simulink model "power_10MW5_diode"  (R2023b)
settings: Solver=FixedStepDiscrete  StartTime=0.0  StopTime=2.6  RelTol=1e-3
InitFcn:
  | power_sysinit
StopFcn:
  | ans = [pl_T1(end),max(tem_T1),pl_T2(end),max(tem_T2),pl_D1(end),max(tem_D1),...
  |     pl_D2(end),max(tem_D2),pl_D5(end),max(tem_D5),i_45(end),i_15(end),pl_D7(end),max(tem_D7)]
values from neighbouring files (symbols this model uses):
  C_absorption = 34e-6    (= 3.4e-05)    [power_sysinit.m]
  f = 40    [power_sysinit.m]
  f_switch = 900    [power_sysinit.m]
  IN = 0.3    [power_sysinit.m]
  L_absorption = 4e-6    (= 4e-06)    [power_sysinit.m]
  m = 1/75*f    (= 0.533333333333)    [power_sysinit.m]
  PM = 0    [power_sysinit.m]
  R_absorption = 0.45    [power_sysinit.m]
  TC = 1/f_switch    (= 0.00111111111111)    [power_sysinit.m]
  temp_init = 40    [power_sysinit.m]
  Ts1 = 1e-6    (= 1e-06)    [power_sysinit.m]
  Ts2 = 500E-6    (= 0.0005)    [power_sysinit.m]
  Udc = 2500    [power_sysinit.m]
undefined symbols (not defined in the file or in its folder): DIODE_204520, DIODE_344520, DIODE_364520, DIODE_364521, DIODE_D1031SH, DIODE_D1331SH, IGCT_364520_36, IGCT_364521_36, IGCT_654522_6, magnitude, Rth_h, Rth_h_tau
libraries: spsMeanLib x138, simulink x32, spsSeriesRLCBranchLib x30, spsRMSLib x24, spsCurrentMeasurementLib x21, dspstat3 x13, spsDiodeLib x12, spsVoltageMeasurementLib x12, spsOnDelayLib x6, powerlib_extras x5, spsDCVoltageSourceLib x4, spsIGBTDiodeLib x4
(part 5 of 6)

== system power_10MW5_diode/JUNCTION LOSS and TEMP/DIODE/36L4521_D/36l4521_MAIN/Subsystem34 ==
  In1 : Inport
  In2 : Inport  Port=2
  In3 : Inport  Port=3
  Abs1 : Abs  SaturateOnIntegerOverflow=off
  Add : Sum
  Constant1 : Constant  Value=0
  Constant2 : Constant  Value=0
  Gain2 : Gain  Gain=Udc/DIODE_364521.Vdc
  Gain3 : Gain  Gain=1/Ts2
  Gain4 : Gain
  Gain8 : Gain  Gain=DIODE_364521.Err/DIODE_364521.IFQ
  Logical Operator1 : Logic  Operator=NOT  AllPortsSameDT=off  OutDataTypeStr=boolean
  Logical Operator11 : Logic  Operator=OR  AllPortsSameDT=off  OutDataTypeStr=boolean
  Logical Operator2 : Logic  Operator=NOT  AllPortsSameDT=off  OutDataTypeStr=boolean
  Logical Operator3 : Logic  AllPortsSameDT=off  OutDataTypeStr=boolean
  Logical Operator4 : Logic  AllPortsSameDT=off  OutDataTypeStr=boolean
  Logical Operator5 : Logic  Operator=NOT  AllPortsSameDT=off  OutDataTypeStr=boolean
  Logical Operator6 : Logic  AllPortsSameDT=off  OutDataTypeStr=boolean
  Pulse Generator : DiscretePulseGenerator  PulseType=Time based  Period=Ts2  PulseWidth=5
  Saturation : Saturate  UpperLimit=5500  LowerLimit=0
  Saturation1 : Saturate  UpperLimit=100  LowerLimit=0
  Scope1 : Scope  NumInputPorts=3
  Scope7 : Scope  NumInputPorts=2
  Switch2 : Switch  Criteria=u2 > Threshold  SaturateOnIntegerOverflow=off  InputSameDT=off
  Switch3 : Switch  Criteria=u2 > Threshold  SaturateOnIntegerOverflow=off  InputSameDT=off
  Switch4 : Switch  Criteria=u2 > Threshold  SaturateOnIntegerOverflow=off  InputSameDT=off
  Unit Delay{,1..4} (5 alike) : UnitDelay  SampleTime=1e-6  HasFrameUpgradeWarning=on
  Out1 : Outport  VectorParamsAs1DForOutWhenUnconnected=off
  wires:
  Abs1/1 -> Add/1
  Switch2/1 -> Gain2/1
  Gain2/1 -> Abs1/1, Scope1/1
  In2/1 -> Logical Operator3/1, Unit Delay/1
  Logical Operator2/1 -> Logical Operator3/2
  Constant2/1 -> Switch2/3
  Switch3/1 -> Add/2
  Constant1/1 -> Switch3/1
  Pulse Generator/1 -> Unit Delay3/1, Logical Operator4/1
  Switch4/1 -> Scope7/2, Gain3/1, Unit Delay2/1
  Unit Delay2/1 -> Switch4/3
  Unit Delay3/1 -> Logical Operator5/1
  Logical Operator5/1 -> Logical Operator4/2
  Logical Operator4/1 -> Switch4/2, Switch3/2, Scope1/3
  Unit Delay1/1 -> Scope7/1, Switch4/1, Switch3/3
  Gain3/1 -> Out1/1
  In1/1 -> Gain4/1
  Add/1 -> Scope1/2, Unit Delay1/1
  Unit Delay/1 -> Logical Operator2/1
  Gain4/1 -> Saturation/1
  Saturation1/1 -> Switch2/1
  In3/1 -> Unit Delay4/1, Logical Operator6/1
  Unit Delay4/1 -> Logical Operator1/1
  Logical Operator6/1 -> Logical Operator11/2
  Logical Operator1/1 -> Logical Operator6/2
  Logical Operator11/1 -> Switch2/2
  Logical Operator3/1 -> Logical Operator11/1
  Saturation/1 -> Gain8/1
  Gain8/1 -> Saturation1/1

== system power_10MW5_diode/JUNCTION LOSS and TEMP/DIODE/36L4521_D/36l4521_MAIN/Subsystem4 ==
  note: 接触热阻：散热器到壳
      | 需考虑单面散热还是双面
      | 时间常数估计的？
  note: 器件手册热阻：壳到结
  note: 散热器热阻：水到壳
  In1 : Inport
  In2 : Inport  Port=2
  Add3 : Sum
  Add4 : Sum  Inputs=5
  Add5 : Sum  Inputs=+++
  Constant : Constant  Value=temp_init
  Discrete Filter1 : DiscreteFilter  Numerator=[Ts2/DIODE_364521.Rth_jc1_dou_tau]  Denominator=[1 (Ts2/DIODE_364521.Rth_jc1_dou_tau)-1]  SampleTime=Ts2
  Discrete Filter2 : DiscreteFilter  Numerator=[Ts2/DIODE_364521.Rth_jc2_dou_tau]  Denominator=[1 (Ts2/DIODE_364521.Rth_jc2_dou_tau)-1]  SampleTime=Ts2
  Discrete Filter3 : DiscreteFilter  Numerator=[Ts2/DIODE_364521.Rth_jc3_dou_tau]  Denominator=[1 (Ts2/DIODE_364521.Rth_jc3_dou_tau)-1]  SampleTime=Ts2
  Discrete Filter4 : DiscreteFilter  Numerator=[Ts2/DIODE_364521.Rth_jc4_dou_tau]  Denominator=[1 (Ts2/DIODE_364521.Rth_jc4_dou_tau)-1]  SampleTime=Ts2
  Discrete Filter5 : DiscreteFilter  Numerator=[Ts2/DIODE_364521.Rth_ch_dou_tau]  Denominator=[1 (Ts2/DIODE_364521.Rth_ch_dou_tau)-1]  SampleTime=Ts2
  Discrete Filter9 : DiscreteFilter  Numerator=[Ts2/Rth_h_tau]  Denominator=[1 (Ts2/Rth_h_tau)-1]  SampleTime=Ts2
  Gain1 : Gain  Gain=DIODE_364521.Rth_jc1_dou
  Gain2 : Gain  Gain=DIODE_364521.Rth_jc2_dou
  Gain3 : Gain  Gain=DIODE_364521.Rth_jc3_dou
  Gain4 : Gain  Gain=DIODE_364521.Rth_jc4_dou
  Gain5 : Gain  Gain=DIODE_364521.Rth_ch_dou
  Gain9 : Gain  Gain=Rth_h
  Out1 : Outport  VectorParamsAs1DForOutWhenUnconnected=off
  wires:
  Discrete Filter9/1 -> Add5/1
  Gain9/1 -> Discrete Filter9/1
  Add3/1 -> Gain2/1, Gain1/1, Gain9/1, Gain4/1, Gain5/1, Gain3/1
  Discrete Filter3/1 -> Add4/4
  Gain3/1 -> Discrete Filter3/1
  Discrete Filter5/1 -> Add4/1
  Gain5/1 -> Discrete Filter5/1
  Discrete Filter1/1 -> Add4/2
  Add5/1 -> Out1/1
  Gain1/1 -> Discrete Filter1/1
  Constant/1 -> Add5/3
  In2/1 -> Add3/2
  Add4/1 -> Add5/2
  Discrete Filter2/1 -> Add4/3
  Gain2/1 -> Discrete Filter2/1
  In1/1 -> Add3/1
  Gain4/1 -> Discrete Filter4/1
  Discrete Filter4/1 -> Add4/5

== system power_10MW5_diode/JUNCTION LOSS and TEMP/DIODE/36L4521_D/36l4521_MAIN/Subsystem5 ==
  In1 : Inport
  Gain44 : Gain  Gain=DIODE_364521.rF
  Gain45 : Gain  Gain=DIODE_364521.VF0
  Math Function9 : Math  Operator=magnitude^2  SignedPower=on
  Mean79 : spsMeanLib/Mean  Freq=2000  Vinit=0  Ts=Ts1
  RMS9 : spsRMSLib/RMS  TrueRMS=on  Freq=2000  RMSInit=0  Ts=Ts1
  Out1 : Outport
  Out2 : Outport  Port=2
  wires:
  Gain45/1 -> Out2/1
  In1/1 -> RMS9/1, Mean79/1
  Math Function9/1 -> Gain44/1
  Mean79/1 -> Gain45/1
  Gain44/1 -> Out1/1
  RMS9/1 -> Math Function9/1

== system power_10MW5_diode/JUNCTION LOSS and TEMP/DIODE/36L4521_D/36l4521_MAIN/Subsystem53 ==
  note: 散热器热阻：水到壳
  note: 器件手册热阻：壳到结
  note: 接触热阻：散热器到壳
      | 需考虑单面散热还是双面
      | 时间常数估计的？
  In1 : Inport
  In2 : Inport  Port=2
  Add3 : Sum
  Add4 : Sum  Inputs=5
  Add5 : Sum  Inputs=+++
  Constant : Constant  Value=temp_init
  Discrete Filter1 : DiscreteFilter  Numerator=[Ts2/DIODE_364521.Rth_jc1_dou_tau]  Denominator=[1 (Ts2/DIODE_364521.Rth_jc1_dou_tau)-1]  SampleTime=Ts2
  Discrete Filter2 : DiscreteFilter  Numerator=[Ts2/DIODE_364521.Rth_jc2_dou_tau]  Denominator=[1 (Ts2/DIODE_364521.Rth_jc2_dou_tau)-1]  SampleTime=Ts2
  Discrete Filter3 : DiscreteFilter  Numerator=[Ts2/DIODE_364521.Rth_jc3_dou_tau]  Denominator=[1 (Ts2/DIODE_364521.Rth_jc3_dou_tau)-1]  SampleTime=Ts2
  Discrete Filter4 : DiscreteFilter  Numerator=[Ts2/DIODE_364521.Rth_jc4_dou_tau]  Denominator=[1 (Ts2/DIODE_364521.Rth_jc4_dou_tau)-1]  SampleTime=Ts2
  Discrete Filter5 : DiscreteFilter  Numerator=[Ts2/DIODE_364521.Rth_ch_dou_tau]  Denominator=[1 (Ts2/DIODE_364521.Rth_ch_dou_tau)-1]  SampleTime=Ts2
  Discrete Filter9 : DiscreteFilter  Numerator=[Ts2/Rth_h_tau]  Denominator=[1 (Ts2/Rth_h_tau)-1]  SampleTime=Ts2
  Gain1 : Gain  Gain=DIODE_364521.Rth_jc1_dou
  Gain2 : Gain  Gain=DIODE_364521.Rth_jc2_dou
  Gain3 : Gain  Gain=DIODE_364521.Rth_jc3_dou
  Gain4 : Gain  Gain=DIODE_364521.Rth_jc4_dou
  Gain5 : Gain  Gain=DIODE_364521.Rth_ch_dou
  Gain9 : Gain  Gain=Rth_h
  Out1 : Outport  VectorParamsAs1DForOutWhenUnconnected=off
  wires:
  Discrete Filter4/1 -> Add4/5
  Gain4/1 -> Discrete Filter4/1
  In1/1 -> Add3/1
  Gain2/1 -> Discrete Filter2/1
  Discrete Filter2/1 -> Add4/3
  Add4/1 -> Add5/2
  In2/1 -> Add3/2
  Constant/1 -> Add5/3
  Gain1/1 -> Discrete Filter1/1
  Add5/1 -> Out1/1
  Discrete Filter1/1 -> Add4/2
  Gain5/1 -> Discrete Filter5/1
  Discrete Filter5/1 -> Add4/1
  Gain3/1 -> Discrete Filter3/1
  Discrete Filter3/1 -> Add4/4
  Add3/1 -> Gain3/1, Gain5/1, Gain4/1, Gain9/1, Gain1/1, Gain2/1
  Gain9/1 -> Discrete Filter9/1
  Discrete Filter9/1 -> Add5/1

== system power_10MW5_diode/JUNCTION LOSS and TEMP/DIODE/36L4521_D/36l4521_MAIN/Subsystem6 ==
  note: 用于判断D1关断时刻，电流为负时，T3开通就意味着D1关断
  In1 : Inport
  In2 : Inport  Port=2
  Abs1 : Abs  SaturateOnIntegerOverflow=off
  Add : Sum
  Constant1 : Constant  Value=0
  Constant2 : Constant  Value=0
  Gain1 : Gain  Gain=Udc/DIODE_364521.Vdc
  Gain2 : Gain  Gain=DIODE_364521.Err/DIODE_364521.IFQ
  Gain3 : Gain  Gain=1/Ts2
  Gain4 : Gain
  Logical Operator2 : Logic  Operator=NOT  AllPortsSameDT=off  OutDataTypeStr=boolean
  Logical Operator3 : Logic  AllPortsSameDT=off  OutDataTypeStr=boolean
  Logical Operator4 : Logic  AllPortsSameDT=off  OutDataTypeStr=boolean
  Logical Operator5 : Logic  Operator=NOT  AllPortsSameDT=off  OutDataTypeStr=boolean
  Pulse Generator : DiscretePulseGenerator  PulseType=Time based  Period=Ts2  PulseWidth=5
  Saturation : Saturate  UpperLimit=5500  LowerLimit=0
  Saturation1 : Saturate  UpperLimit=100  LowerLimit=0
  Switch2 : Switch  Criteria=u2 > Threshold  SaturateOnIntegerOverflow=off  InputSameDT=off
  Switch3 : Switch  Criteria=u2 > Threshold  SaturateOnIntegerOverflow=off  InputSameDT=off
  Switch4 : Switch  Criteria=u2 > Threshold  SaturateOnIntegerOverflow=off  InputSameDT=off
  Unit Delay{,1..3} (4 alike) : UnitDelay  SampleTime=Ts1  HasFrameUpgradeWarning=on
  Out1 : Outport  VectorParamsAs1DForOutWhenUnconnected=off
  wires:
  Gain2/1 -> Saturation1/1
  Saturation/1 -> Gain2/1
  Saturation1/1 -> Switch2/1
  Gain4/1 -> Saturation/1
  Unit Delay/1 -> Logical Operator2/1
  Add/1 -> Unit Delay1/1
  In1/1 -> Gain4/1
  Gain3/1 -> Out1/1
  Unit Delay1/1 -> Switch4/1, Switch3/3
  Logical Operator4/1 -> Switch3/2, Switch4/2
  Logical Operator5/1 -> Logical Operator4/2
  Unit Delay3/1 -> Logical Operator5/1
  Unit Delay2/1 -> Switch4/3
  Switch4/1 -> Gain3/1, Unit Delay2/1
  Pulse Generator/1 -> Logical Operator4/1, Unit Delay3/1
  Constant1/1 -> Switch3/1
  Switch3/1 -> Add/2
  Constant2/1 -> Switch2/3
  Logical Operator3/1 -> Switch2/2
  Logical Operator2/1 -> Logical Operator3/2
  In2/1 -> Unit Delay/1, Logical Operator3/1
  Gain1/1 -> Abs1/1
  Switch2/1 -> Gain1/1
  Abs1/1 -> Add/1

== system power_10MW5_diode/JUNCTION LOSS and TEMP/DIODE/36L4521_D/36l4521_MAIN/Subsystem7 ==
  note: 散热器热阻：水到壳
  note: 器件手册热阻：壳到结
  note: 接触热阻：散热器到壳
      | 需考虑单面散热还是双面
      | 时间常数估计的？
  In1 : Inport
  In2 : Inport  Port=2
  Add3 : Sum
  Add4 : Sum  Inputs=5
  Add5 : Sum  Inputs=+++
  Constant : Constant  Value=temp_init
  Discrete Filter1 : DiscreteFilter  Numerator=[Ts2/DIODE_364521.Rth_jc1_dou_tau]  Denominator=[1 (Ts2/DIODE_364521.Rth_jc1_dou_tau)-1]  SampleTime=Ts2
  Discrete Filter2 : DiscreteFilter  Numerator=[Ts2/DIODE_364521.Rth_jc2_dou_tau]  Denominator=[1 (Ts2/DIODE_364521.Rth_jc2_dou_tau)-1]  SampleTime=Ts2
  Discrete Filter3 : DiscreteFilter  Numerator=[Ts2/DIODE_364521.Rth_jc3_dou_tau]  Denominator=[1 (Ts2/DIODE_364521.Rth_jc3_dou_tau)-1]  SampleTime=Ts2
  Discrete Filter4 : DiscreteFilter  Numerator=[Ts2/DIODE_364521.Rth_jc4_dou_tau]  Denominator=[1 (Ts2/DIODE_364521.Rth_jc4_dou_tau)-1]  SampleTime=Ts2
  Discrete Filter5 : DiscreteFilter  Numerator=[Ts2/DIODE_364521.Rth_ch_dou_tau]  Denominator=[1 (Ts2/DIODE_364521.Rth_ch_dou_tau)-1]  SampleTime=Ts2
  Discrete Filter9 : DiscreteFilter  Numerator=[Ts2/Rth_h_tau]  Denominator=[1 (Ts2/Rth_h_tau)-1]  SampleTime=Ts2
  Gain1 : Gain  Gain=DIODE_364521.Rth_jc1_dou
  Gain2 : Gain  Gain=DIODE_364521.Rth_jc2_dou
  Gain3 : Gain  Gain=DIODE_364521.Rth_jc3_dou
  Gain4 : Gain  Gain=DIODE_364521.Rth_jc4_dou
  Gain5 : Gain  Gain=DIODE_364521.Rth_ch_dou
  Gain9 : Gain  Gain=Rth_h
  Out1 : Outport  VectorParamsAs1DForOutWhenUnconnected=off
  wires:
  Discrete Filter4/1 -> Add4/5
  Gain4/1 -> Discrete Filter4/1
  In1/1 -> Add3/1
  Gain2/1 -> Discrete Filter2/1
  Discrete Filter2/1 -> Add4/3
  Add4/1 -> Add5/2
  In2/1 -> Add3/2
  Constant/1 -> Add5/3
  Gain1/1 -> Discrete Filter1/1
  Add5/1 -> Out1/1
  Discrete Filter1/1 -> Add4/2
  Gain5/1 -> Discrete Filter5/1
  Discrete Filter5/1 -> Add4/1
  Gain3/1 -> Discrete Filter3/1
  Discrete Filter3/1 -> Add4/4
  Add3/1 -> Gain3/1, Gain5/1, Gain4/1, Gain9/1, Gain1/1, Gain2/1
  Gain9/1 -> Discrete Filter9/1
  Discrete Filter9/1 -> Add5/1

== system power_10MW5_diode/JUNCTION LOSS and TEMP/DIODE/36L4521_D/36l4521_MAIN/Subsystem8 ==
  In1 : Inport
  Gain44 : Gain  Gain=DIODE_364521.rF
  Gain45 : Gain  Gain=DIODE_364521.VF0
  Math Function9 : Math  Operator=magnitude^2  SignedPower=on
  Mean79 : spsMeanLib/Mean  Freq=2000  Vinit=0  Ts=Ts1
  RMS9 : spsRMSLib/RMS  TrueRMS=on  Freq=2000  RMSInit=0  Ts=Ts1
  Out1 : Outport
  Out2 : Outport  Port=2
  wires:
  RMS9/1 -> Math Function9/1
  Gain44/1 -> Out1/1
  Mean79/1 -> Gain45/1
  Math Function9/1 -> Gain44/1
  In1/1 -> Mean79/1, RMS9/1
  Gain45/1 -> Out2/1

== system power_10MW5_diode/JUNCTION LOSS and TEMP/DIODE/D1031SH/D1031SH_MAIN/Subsystem ==
  In1 : Inport
  Gain44 : Gain  Gain=DIODE_D1031SH.rF
  Gain45 : Gain  Gain=DIODE_D1031SH.VF0
  Math Function9 : Math  Operator=magnitude^2  SignedPower=on
  Mean79 : spsMeanLib/Mean  Freq=2000  Vinit=0  Ts=Ts1
  RMS9 : spsRMSLib/RMS  TrueRMS=on  Freq=2000  RMSInit=0  Ts=Ts1
  Out1 : Outport
  Out2 : Outport  Port=2
  wires:
  RMS9/1 -> Math Function9/1
  Gain44/1 -> Out1/1
  Mean79/1 -> Gain45/1
  Math Function9/1 -> Gain44/1
  In1/1 -> Mean79/1, RMS9/1
  Gain45/1 -> Out2/1

== system power_10MW5_diode/JUNCTION LOSS and TEMP/DIODE/D1031SH/D1031SH_MAIN/Subsystem1 ==
  note: 接触热阻：散热器到壳
      | 需考虑单面散热还是双面
      | 时间常数估计的？
  note: 器件手册热阻：壳到结
  note: 散热器热阻：水到壳
  In1 : Inport
  In2 : Inport  Port=2
  Add3 : Sum
  Add4 : Sum  Inputs=6
  Add5 : Sum  Inputs=+++
  Constant : Constant  Value=temp_init
  Discrete Filter1 : DiscreteFilter  Numerator=[Ts2/DIODE_D1031SH.Rth_jc1_dou_tau]  Denominator=[1 (Ts2/DIODE_D1031SH.Rth_jc1_dou_tau)-1]  SampleTime=Ts2
  Discrete Filter2 : DiscreteFilter  Numerator=[Ts2/DIODE_D1031SH.Rth_jc2_dou_tau]  Denominator=[1 (Ts2/DIODE_D1031SH.Rth_jc2_dou_tau)-1]  SampleTime=Ts2
  Discrete Filter3 : DiscreteFilter  Numerator=[Ts2/DIODE_D1031SH.Rth_jc3_dou_tau]  Denominator=[1 (Ts2/DIODE_D1031SH.Rth_jc3_dou_tau)-1]  SampleTime=Ts2
  Discrete Filter4 : DiscreteFilter  Numerator=[Ts2/DIODE_D1031SH.Rth_jc4_dou_tau]  Denominator=[1 (Ts2/DIODE_D1031SH.Rth_jc4_dou_tau)-1]  SampleTime=Ts2
  Discrete Filter5 : DiscreteFilter  Numerator=[Ts2/DIODE_D1031SH.Rth_ch_dou_tau]  Denominator=[1 (Ts2/DIODE_D1031SH.Rth_ch_dou_tau)-1]  SampleTime=Ts2
  Discrete Filter6 : DiscreteFilter  Numerator=[Ts2/DIODE_D1031SH.Rth_jc5_dou_tau]  Denominator=[1 (Ts2/DIODE_D1031SH.Rth_jc5_dou_tau)-1]  SampleTime=Ts2
  Discrete Filter9 : DiscreteFilter  Numerator=[Ts2/Rth_h_tau]  Denominator=[1 (Ts2/Rth_h_tau)-1]  SampleTime=Ts2
  Gain1 : Gain  Gain=DIODE_D1031SH.Rth_jc1_dou
  Gain2 : Gain  Gain=DIODE_D1031SH.Rth_jc2_dou
  Gain3 : Gain  Gain=DIODE_D1031SH.Rth_jc3_dou
  Gain4 : Gain  Gain=DIODE_D1031SH.Rth_jc4_dou
  Gain5 : Gain  Gain=DIODE_D1031SH.Rth_ch_dou
  Gain6 : Gain  Gain=DIODE_D1031SH.Rth_jc5_dou
  Gain9 : Gain  Gain=Rth_h
  Out1 : Outport  VectorParamsAs1DForOutWhenUnconnected=off
  wires:
  Discrete Filter6/1 -> Add4/6
  Gain6/1 -> Discrete Filter6/1
  Discrete Filter9/1 -> Add5/1
  Gain9/1 -> Discrete Filter9/1
  Add3/1 -> Gain2/1, Gain1/1, Gain9/1, Gain4/1, Gain6/1, Gain5/1, Gain3/1
  Discrete Filter3/1 -> Add4/4
  Gain3/1 -> Discrete Filter3/1
  Discrete Filter5/1 -> Add4/1
  Gain5/1 -> Discrete Filter5/1
  Discrete Filter1/1 -> Add4/2
  Add5/1 -> Out1/1
  Gain1/1 -> Discrete Filter1/1
  Constant/1 -> Add5/3
  In2/1 -> Add3/2
  Add4/1 -> Add5/2
  Discrete Filter2/1 -> Add4/3
  Gain2/1 -> Discrete Filter2/1
  In1/1 -> Add3/1
  Gain4/1 -> Discrete Filter4/1
  Discrete Filter4/1 -> Add4/5

== system power_10MW5_diode/JUNCTION LOSS and TEMP/DIODE/D1031SH/D1031SH_MAIN/Subsystem2 ==
  In1 : Inport
  Gain44 : Gain  Gain=DIODE_D1031SH.rF
  Gain45 : Gain  Gain=DIODE_D1031SH.VF0
  Math Function9 : Math  Operator=magnitude^2  SignedPower=on
  Mean79 : spsMeanLib/Mean  Freq=2000  Vinit=0  Ts=Ts1
  RMS9 : spsRMSLib/RMS  TrueRMS=on  Freq=2000  RMSInit=0  Ts=Ts1
  Out1 : Outport
  Out2 : Outport  Port=2
  wires:
  Gain45/1 -> Out2/1
  In1/1 -> RMS9/1, Mean79/1
  Math Function9/1 -> Gain44/1
  Mean79/1 -> Gain45/1
  Gain44/1 -> Out1/1
  RMS9/1 -> Math Function9/1

== system power_10MW5_diode/JUNCTION LOSS and TEMP/DIODE/D1031SH/D1031SH_MAIN/Subsystem29 ==
  note: 用于判断D1关断时刻，电流为负时，T3开通就意味着D1关断
  In1 : Inport
  In2 : Inport  Port=2
  Abs1 : Abs  SaturateOnIntegerOverflow=off
  Add : Sum
  Constant1 : Constant  Value=0
  Constant2 : Constant  Value=0
  Gain1 : Gain  Gain=Udc/DIODE_D1031SH.Vdc
  Gain2 : Gain  Gain=DIODE_D1031SH.Err/DIODE_D1031SH.IFQ
  Gain3 : Gain  Gain=1/Ts2
  Gain4 : Gain
  Logical Operator2 : Logic  Operator=NOT  AllPortsSameDT=off  OutDataTypeStr=boolean
  Logical Operator3 : Logic  AllPortsSameDT=off  OutDataTypeStr=boolean
  Logical Operator4 : Logic  AllPortsSameDT=off  OutDataTypeStr=boolean
  Logical Operator5 : Logic  Operator=NOT  AllPortsSameDT=off  OutDataTypeStr=boolean
  Pulse Generator : DiscretePulseGenerator  PulseType=Time based  Period=Ts2  PulseWidth=5
  Saturation : Saturate  UpperLimit=5500  LowerLimit=0
  Saturation1 : Saturate  UpperLimit=100  LowerLimit=0
  Switch2 : Switch  Criteria=u2 > Threshold  SaturateOnIntegerOverflow=off  InputSameDT=off
  Switch3 : Switch  Criteria=u2 > Threshold  SaturateOnIntegerOverflow=off  InputSameDT=off
  Switch4 : Switch  Criteria=u2 > Threshold  SaturateOnIntegerOverflow=off  InputSameDT=off
  Unit Delay{,1..3} (4 alike) : UnitDelay  SampleTime=Ts1  HasFrameUpgradeWarning=on
  Out1 : Outport  VectorParamsAs1DForOutWhenUnconnected=off
  wires:
  Abs1/1 -> Add/1
  Switch2/1 -> Gain1/1
  Gain1/1 -> Abs1/1
  In2/1 -> Logical Operator3/1, Unit Delay/1
  Logical Operator2/1 -> Logical Operator3/2
  Logical Operator3/1 -> Switch2/2
  Constant2/1 -> Switch2/3
  Switch3/1 -> Add/2
  Constant1/1 -> Switch3/1
  Pulse Generator/1 -> Unit Delay3/1, Logical Operator4/1
  Switch4/1 -> Unit Delay2/1, Gain3/1
  Unit Delay2/1 -> Switch4/3
  Unit Delay3/1 -> Logical Operator5/1
  Logical Operator5/1 -> Logical Operator4/2
  Logical Operator4/1 -> Switch4/2, Switch3/2
  Unit Delay1/1 -> Switch3/3, Switch4/1
  Gain3/1 -> Out1/1
  In1/1 -> Gain4/1
  Add/1 -> Unit Delay1/1
  Unit Delay/1 -> Logical Operator2/1
  Gain4/1 -> Saturation/1
  Saturation1/1 -> Switch2/1
  Saturation/1 -> Gain2/1
  Gain2/1 -> Saturation1/1

== system power_10MW5_diode/JUNCTION LOSS and TEMP/DIODE/D1031SH/D1031SH_MAIN/Subsystem3 ==
  In1 : Inport
  Abs1 : Abs  SaturateOnIntegerOverflow=off
  Add : Sum
  Add1 : Sum
  Constant : Constant
  Constant1 : Constant  Value=0
  Constant2 : Constant  Value=0
  Data Type Conversion : DataTypeConversion  OutDataTypeStr=boolean  SaturateOnIntegerOverflow=off  RndMeth=Floor
  Data Type Conversion1 : DataTypeConversion  SaturateOnIntegerOverflow=off  RndMeth=Floor
  Gain : Gain  Gain=-1
  Gain2 : Gain  Gain=Udc/DIODE_D1031SH.Vdc
  Gain3 : Gain  Gain=1/Ts2
  Gain6 : Gain
  Gain8 : Gain  Gain=DIODE_D1031SH.Err/DIODE_D1031SH.IFQ
  Logical Operator2 : Logic  Operator=NOT  AllPortsSameDT=off  OutDataTypeStr=boolean
  Logical Operator4 : Logic  AllPortsSameDT=off  OutDataTypeStr=boolean
  Logical Operator5 : Logic  Operator=NOT  AllPortsSameDT=off  OutDataTypeStr=boolean
  Pulse Generator : DiscretePulseGenerator  PulseType=Time based  Period=Ts2  PulseWidth=5
  Saturation2 : Saturate  UpperLimit=5500  LowerLimit=0
  Saturation3 : Saturate  UpperLimit=100  LowerLimit=0
  Scope1 : Scope  NumInputPorts=3
  Scope7 : Scope  NumInputPorts=2
  Switch2 : Switch  Criteria=u2 > Threshold  Threshold=-1  SaturateOnIntegerOverflow=off  InputSameDT=off
  Switch3 : Switch  Criteria=u2 > Threshold  SaturateOnIntegerOverflow=off  InputSameDT=off
  Switch4 : Switch  Criteria=u2 > Threshold  SaturateOnIntegerOverflow=off  InputSameDT=off
  Terminator : Terminator
  Unit Delay{,1..3} (4 alike) : UnitDelay  SampleTime=1e-6  HasFrameUpgradeWarning=on
  Out1 : Outport  VectorParamsAs1DForOutWhenUnconnected=off
  wires:
  Add/1 -> Unit Delay1/1, Scope1/2
  Gain3/1 -> Out1/1
  Unit Delay1/1 -> Switch4/1, Switch3/3, Scope7/1
  Logical Operator4/1 -> Switch3/2, Switch4/2, Scope1/3
  Logical Operator5/1 -> Logical Operator4/2
  Unit Delay3/1 -> Logical Operator5/1
  Unit Delay2/1 -> Switch4/3
  Switch4/1 -> Gain3/1, Unit Delay2/1, Scope7/2
  Pulse Generator/1 -> Logical Operator4/1, Unit Delay3/1
  Constant1/1 -> Switch3/1
  Switch3/1 -> Add/2
  Constant2/1 -> Switch2/3
  In1/1 -> Data Type Conversion/1, Gain6/1
  Gain2/1 -> Scope1/1, Abs1/1
  Switch2/1 -> Gain2/1
  Abs1/1 -> Add/1
  Unit Delay/1 -> Logical Operator2/1
  Logical Operator2/1 -> Add1/2
  Data Type Conversion/1 -> Add1/1, Unit Delay/1
  Add1/1 -> Data Type Conversion1/1
  Gain/1 -> Switch2/2
  Data Type Conversion1/1 -> Gain/1
  Constant/1 -> Switch2/1
  Gain6/1 -> Saturation2/1
  Saturation2/1 -> Gain8/1
  Gain8/1 -> Saturation3/1
  Saturation3/1 -> Terminator/1

== system power_10MW5_diode/JUNCTION LOSS and TEMP/DIODE/D1031SH/D1031SH_MAIN/Subsystem34 ==
  In1 : Inport
  In2 : Inport  Port=2
  In3 : Inport  Port=3
  Abs1 : Abs  SaturateOnIntegerOverflow=off
  Add : Sum
  Constant1 : Constant  Value=0
  Constant2 : Constant  Value=0
  Gain2 : Gain  Gain=Udc/DIODE_204520.Vdc
  Gain3 : Gain  Gain=1/Ts2
  Gain4 : Gain
  Gain8 : Gain  Gain=DIODE_D1031SH.Err/DIODE_D1031SH.IFQ
  Logical Operator1 : Logic  Operator=NOT  AllPortsSameDT=off  OutDataTypeStr=boolean
  Logical Operator11 : Logic  Operator=OR  AllPortsSameDT=off  OutDataTypeStr=boolean
  Logical Operator2 : Logic  Operator=NOT  AllPortsSameDT=off  OutDataTypeStr=boolean
  Logical Operator3 : Logic  AllPortsSameDT=off  OutDataTypeStr=boolean
  Logical Operator4 : Logic  AllPortsSameDT=off  OutDataTypeStr=boolean
  Logical Operator5 : Logic  Operator=NOT  AllPortsSameDT=off  OutDataTypeStr=boolean
  Logical Operator6 : Logic  AllPortsSameDT=off  OutDataTypeStr=boolean
  Pulse Generator : DiscretePulseGenerator  PulseType=Time based  Period=Ts2  PulseWidth=5
  Saturation : Saturate  UpperLimit=5500  LowerLimit=0
  Saturation1 : Saturate  UpperLimit=100  LowerLimit=0
  Scope1 : Scope  NumInputPorts=3
  Scope7 : Scope  NumInputPorts=2
  Switch2 : Switch  Criteria=u2 > Threshold  SaturateOnIntegerOverflow=off  InputSameDT=off
  Switch3 : Switch  Criteria=u2 > Threshold  SaturateOnIntegerOverflow=off  InputSameDT=off
  Switch4 : Switch  Criteria=u2 > Threshold  SaturateOnIntegerOverflow=off  InputSameDT=off
  Unit Delay{,1..4} (5 alike) : UnitDelay  SampleTime=1e-6  HasFrameUpgradeWarning=on
  Out1 : Outport  VectorParamsAs1DForOutWhenUnconnected=off
  wires:
  Abs1/1 -> Add/1
  Switch2/1 -> Gain2/1
  Gain2/1 -> Abs1/1, Scope1/1
  In2/1 -> Logical Operator3/1, Unit Delay/1
  Logical Operator2/1 -> Logical Operator3/2
  Constant2/1 -> Switch2/3
  Switch3/1 -> Add/2
  Constant1/1 -> Switch3/1
  Pulse Generator/1 -> Unit Delay3/1, Logical Operator4/1
  Switch4/1 -> Scope7/2, Gain3/1, Unit Delay2/1
  Unit Delay2/1 -> Switch4/3
  Unit Delay3/1 -> Logical Operator5/1
  Logical Operator5/1 -> Logical Operator4/2
  Logical Operator4/1 -> Switch4/2, Switch3/2, Scope1/3
  Unit Delay1/1 -> Scope7/1, Switch4/1, Switch3/3
  Gain3/1 -> Out1/1
  In1/1 -> Gain4/1
  Add/1 -> Scope1/2, Unit Delay1/1
  Unit Delay/1 -> Logical Operator2/1
  Gain4/1 -> Saturation/1
  Saturation1/1 -> Switch2/1
  In3/1 -> Unit Delay4/1, Logical Operator6/1
  Unit Delay4/1 -> Logical Operator1/1
  Logical Operator6/1 -> Logical Operator11/2
  Logical Operator1/1 -> Logical Operator6/2
  Logical Operator11/1 -> Switch2/2
  Logical Operator3/1 -> Logical Operator11/1
  Saturation/1 -> Gain8/1
  Gain8/1 -> Saturation1/1

== system power_10MW5_diode/JUNCTION LOSS and TEMP/DIODE/D1031SH/D1031SH_MAIN/Subsystem4 ==
  note: 接触热阻：散热器到壳
      | 需考虑单面散热还是双面
      | 时间常数估计的？
  note: 器件手册热阻：壳到结
  note: 散热器热阻：水到壳
  In1 : Inport
  In2 : Inport  Port=2
  Add3 : Sum
  Add4 : Sum  Inputs=6
  Add5 : Sum  Inputs=+++
  Constant : Constant  Value=temp_init
  Discrete Filter1 : DiscreteFilter  Numerator=[Ts2/DIODE_D1031SH.Rth_jc1_dou_tau]  Denominator=[1 (Ts2/DIODE_D1031SH.Rth_jc1_dou_tau)-1]  SampleTime=Ts2
  Discrete Filter2 : DiscreteFilter  Numerator=[Ts2/DIODE_D1031SH.Rth_jc2_dou_tau]  Denominator=[1 (Ts2/DIODE_D1031SH.Rth_jc2_dou_tau)-1]  SampleTime=Ts2
  Discrete Filter3 : DiscreteFilter  Numerator=[Ts2/DIODE_D1031SH.Rth_jc3_dou_tau]  Denominator=[1 (Ts2/DIODE_D1031SH.Rth_jc3_dou_tau)-1]  SampleTime=Ts2
  Discrete Filter4 : DiscreteFilter  Numerator=[Ts2/DIODE_D1031SH.Rth_jc4_dou_tau]  Denominator=[1 (Ts2/DIODE_D1031SH.Rth_jc4_dou_tau)-1]  SampleTime=Ts2
  Discrete Filter5 : DiscreteFilter  Numerator=[Ts2/DIODE_D1031SH.Rth_ch_dou_tau]  Denominator=[1 (Ts2/DIODE_D1031SH.Rth_ch_dou_tau)-1]  SampleTime=Ts2
  Discrete Filter6 : DiscreteFilter  Numerator=[Ts2/DIODE_D1031SH.Rth_jc5_dou_tau]  Denominator=[1 (Ts2/DIODE_D1031SH.Rth_jc5_dou_tau)-1]  SampleTime=Ts2
  Discrete Filter9 : DiscreteFilter  Numerator=[Ts2/Rth_h_tau]  Denominator=[1 (Ts2/Rth_h_tau)-1]  SampleTime=Ts2
  Gain1 : Gain  Gain=DIODE_D1031SH.Rth_jc1_dou
  Gain2 : Gain  Gain=DIODE_D1031SH.Rth_jc2_dou
  Gain3 : Gain  Gain=DIODE_D1031SH.Rth_jc3_dou
  Gain4 : Gain  Gain=DIODE_D1031SH.Rth_jc4_dou
  Gain5 : Gain  Gain=DIODE_D1031SH.Rth_ch_dou
  Gain6 : Gain  Gain=DIODE_D1031SH.Rth_jc5_dou
  Gain9 : Gain  Gain=Rth_h
  Out1 : Outport  VectorParamsAs1DForOutWhenUnconnected=off
  wires:
  Discrete Filter6/1 -> Add4/6
  Gain6/1 -> Discrete Filter6/1
  Discrete Filter9/1 -> Add5/1
  Gain9/1 -> Discrete Filter9/1
  Add3/1 -> Gain2/1, Gain1/1, Gain9/1, Gain4/1, Gain6/1, Gain5/1, Gain3/1
  Discrete Filter3/1 -> Add4/4
  Gain3/1 -> Discrete Filter3/1
  Discrete Filter5/1 -> Add4/1
  Gain5/1 -> Discrete Filter5/1
  Discrete Filter1/1 -> Add4/2
  Add5/1 -> Out1/1
  Gain1/1 -> Discrete Filter1/1
  Constant/1 -> Add5/3
  In2/1 -> Add3/2
  Add4/1 -> Add5/2
  Discrete Filter2/1 -> Add4/3
  Gain2/1 -> Discrete Filter2/1
  In1/1 -> Add3/1
  Gain4/1 -> Discrete Filter4/1
  Discrete Filter4/1 -> Add4/5

== system power_10MW5_diode/JUNCTION LOSS and TEMP/DIODE/D1031SH/D1031SH_MAIN/Subsystem5 ==
  In1 : Inport
  Gain44 : Gain  Gain=DIODE_D1031SH.rF
  Gain45 : Gain  Gain=DIODE_D1031SH.VF0
  Math Function9 : Math  Operator=magnitude^2  SignedPower=on
  Mean79 : spsMeanLib/Mean  Freq=2000  Vinit=0  Ts=Ts1
  RMS9 : spsRMSLib/RMS  TrueRMS=on  Freq=2000  RMSInit=0  Ts=Ts1
  Out1 : Outport
  Out2 : Outport  Port=2
  wires:
  RMS9/1 -> Math Function9/1
  Gain44/1 -> Out1/1
  Mean79/1 -> Gain45/1
  Math Function9/1 -> Gain44/1
  In1/1 -> Mean79/1, RMS9/1
  Gain45/1 -> Out2/1

== system power_10MW5_diode/JUNCTION LOSS and TEMP/DIODE/D1031SH/D1031SH_MAIN/Subsystem53 ==
  note: 散热器热阻：水到壳
  note: 器件手册热阻：壳到结
  note: 接触热阻：散热器到壳
      | 需考虑单面散热还是双面
      | 时间常数估计的？
  In1 : Inport
  In2 : Inport  Port=2
  Add3 : Sum
  Add4 : Sum  Inputs=6
  Add5 : Sum  Inputs=+++
  Constant : Constant  Value=temp_init
  Discrete Filter1 : DiscreteFilter  Numerator=[Ts2/DIODE_D1031SH.Rth_jc1_dou_tau]  Denominator=[1 (Ts2/DIODE_D1031SH.Rth_jc1_dou_tau)-1]  SampleTime=Ts2
  Discrete Filter2 : DiscreteFilter  Numerator=[Ts2/DIODE_D1031SH.Rth_jc2_dou_tau]  Denominator=[1 (Ts2/DIODE_D1031SH.Rth_jc2_dou_tau)-1]  SampleTime=Ts2
  Discrete Filter3 : DiscreteFilter  Numerator=[Ts2/DIODE_D1031SH.Rth_jc3_dou_tau]  Denominator=[1 (Ts2/DIODE_D1031SH.Rth_jc3_dou_tau)-1]  SampleTime=Ts2
  Discrete Filter4 : DiscreteFilter  Numerator=[Ts2/DIODE_D1031SH.Rth_jc4_dou_tau]  Denominator=[1 (Ts2/DIODE_D1031SH.Rth_jc4_dou_tau)-1]  SampleTime=Ts2
  Discrete Filter5 : DiscreteFilter  Numerator=[Ts2/DIODE_D1031SH.Rth_ch_dou_tau]  Denominator=[1 (Ts2/DIODE_D1031SH.Rth_ch_dou_tau)-1]  SampleTime=Ts2
  Discrete Filter6 : DiscreteFilter  Numerator=[Ts2/DIODE_D1031SH.Rth_jc5_dou_tau]  Denominator=[1 (Ts2/DIODE_D1031SH.Rth_jc5_dou_tau)-1]  SampleTime=Ts2
  Discrete Filter9 : DiscreteFilter  Numerator=[Ts2/Rth_h_tau]  Denominator=[1 (Ts2/Rth_h_tau)-1]  SampleTime=Ts2
  Gain1 : Gain  Gain=DIODE_D1031SH.Rth_jc1_dou
  Gain2 : Gain  Gain=DIODE_D1031SH.Rth_jc2_dou
  Gain3 : Gain  Gain=DIODE_D1031SH.Rth_jc3_dou
  Gain4 : Gain  Gain=DIODE_D1031SH.Rth_jc4_dou
  Gain5 : Gain  Gain=DIODE_D1031SH.Rth_ch_dou
  Gain6 : Gain  Gain=DIODE_D1031SH.Rth_jc5_dou
  Gain9 : Gain  Gain=Rth_h
  Out1 : Outport  VectorParamsAs1DForOutWhenUnconnected=off
  wires:
  Discrete Filter4/1 -> Add4/5
  Gain4/1 -> Discrete Filter4/1
  In1/1 -> Add3/1
  Gain2/1 -> Discrete Filter2/1
  Discrete Filter2/1 -> Add4/3
  Add4/1 -> Add5/2
  In2/1 -> Add3/2
  Constant/1 -> Add5/3
  Gain1/1 -> Discrete Filter1/1
  Add5/1 -> Out1/1
  Discrete Filter1/1 -> Add4/2
  Gain5/1 -> Discrete Filter5/1
  Discrete Filter5/1 -> Add4/1
  Gain3/1 -> Discrete Filter3/1
  Discrete Filter3/1 -> Add4/4
  Add3/1 -> Gain3/1, Gain5/1, Gain6/1, Gain4/1, Gain9/1, Gain1/1, Gain2/1
  Gain9/1 -> Discrete Filter9/1
  Discrete Filter9/1 -> Add5/1
  Gain6/1 -> Discrete Filter6/1
  Discrete Filter6/1 -> Add4/6

== system power_10MW5_diode/JUNCTION LOSS and TEMP/DIODE/D1031SH/D1031SH_MAIN/Subsystem6 ==
  note: 散热器热阻：水到壳
  note: 器件手册热阻：壳到结
  note: 接触热阻：散热器到壳
      | 需考虑单面散热还是双面
      | 时间常数估计的？
  In1 : Inport
  In2 : Inport  Port=2
  Add3 : Sum
  Add4 : Sum  Inputs=6
  Add5 : Sum  Inputs=+++
  Constant : Constant  Value=temp_init
  Discrete Filter1 : DiscreteFilter  Numerator=[Ts2/DIODE_D1031SH.Rth_jc1_dou_tau]  Denominator=[1 (Ts2/DIODE_D1031SH.Rth_jc1_dou_tau)-1]  SampleTime=Ts2
  Discrete Filter2 : DiscreteFilter  Numerator=[Ts2/DIODE_D1031SH.Rth_jc2_dou_tau]  Denominator=[1 (Ts2/DIODE_D1031SH.Rth_jc2_dou_tau)-1]  SampleTime=Ts2
  Discrete Filter3 : DiscreteFilter  Numerator=[Ts2/DIODE_D1031SH.Rth_jc3_dou_tau]  Denominator=[1 (Ts2/DIODE_D1031SH.Rth_jc3_dou_tau)-1]  SampleTime=Ts2
  Discrete Filter4 : DiscreteFilter  Numerator=[Ts2/DIODE_D1031SH.Rth_jc4_dou_tau]  Denominator=[1 (Ts2/DIODE_D1031SH.Rth_jc4_dou_tau)-1]  SampleTime=Ts2
  Discrete Filter5 : DiscreteFilter  Numerator=[Ts2/DIODE_D1031SH.Rth_ch_dou_tau]  Denominator=[1 (Ts2/DIODE_D1031SH.Rth_ch_dou_tau)-1]  SampleTime=Ts2
  Discrete Filter6 : DiscreteFilter  Numerator=[Ts2/DIODE_D1031SH.Rth_jc5_dou_tau]  Denominator=[1 (Ts2/DIODE_D1031SH.Rth_jc5_dou_tau)-1]  SampleTime=Ts2
  Discrete Filter9 : DiscreteFilter  Numerator=[Ts2/Rth_h_tau]  Denominator=[1 (Ts2/Rth_h_tau)-1]  SampleTime=Ts2
  Gain1 : Gain  Gain=DIODE_D1031SH.Rth_jc1_dou
  Gain2 : Gain  Gain=DIODE_D1031SH.Rth_jc2_dou
  Gain3 : Gain  Gain=DIODE_D1031SH.Rth_jc3_dou
  Gain4 : Gain  Gain=DIODE_D1031SH.Rth_jc4_dou
  Gain5 : Gain  Gain=DIODE_D1031SH.Rth_ch_dou
  Gain6 : Gain  Gain=DIODE_D1031SH.Rth_jc5_dou
  Gain9 : Gain  Gain=Rth_h
  Out1 : Outport  VectorParamsAs1DForOutWhenUnconnected=off
  wires:
  Discrete Filter4/1 -> Add4/5
  Gain4/1 -> Discrete Filter4/1
  In1/1 -> Add3/1
  Gain2/1 -> Discrete Filter2/1
  Discrete Filter2/1 -> Add4/3
  Add4/1 -> Add5/2
  In2/1 -> Add3/2
  Constant/1 -> Add5/3
  Gain1/1 -> Discrete Filter1/1
  Add5/1 -> Out1/1
  Discrete Filter1/1 -> Add4/2
  Gain5/1 -> Discrete Filter5/1
  Discrete Filter5/1 -> Add4/1
  Gain3/1 -> Discrete Filter3/1
  Discrete Filter3/1 -> Add4/4
  Add3/1 -> Gain3/1, Gain5/1, Gain6/1, Gain4/1, Gain9/1, Gain1/1, Gain2/1
  Gain9/1 -> Discrete Filter9/1
  Discrete Filter9/1 -> Add5/1
  Gain6/1 -> Discrete Filter6/1
  Discrete Filter6/1 -> Add4/6

== system power_10MW5_diode/JUNCTION LOSS and TEMP/DIODE/D1031SH/D1031SH_MAIN/Subsystem7 ==
  In1 : Inport
  Gain44 : Gain  Gain=DIODE_D1031SH.rF
  Gain45 : Gain  Gain=DIODE_D1031SH.VF0
  Math Function9 : Math  Operator=magnitude^2  SignedPower=on
  Mean79 : spsMeanLib/Mean  Freq=2000  Vinit=0  Ts=Ts1
  RMS9 : spsRMSLib/RMS  TrueRMS=on  Freq=2000  RMSInit=0  Ts=Ts1
  Out1 : Outport
  Out2 : Outport  Port=2
  wires:
  Gain45/1 -> Out2/1
  In1/1 -> RMS9/1, Mean79/1
  Math Function9/1 -> Gain44/1
  Mean79/1 -> Gain45/1
  Gain44/1 -> Out1/1
  RMS9/1 -> Math Function9/1

== system power_10MW5_diode/JUNCTION LOSS and TEMP/DIODE/D1031SH/D1031SH_MAIN/Subsystem9 ==
  note: 用于判断D1关断时刻，电流为负时，T3开通就意味着D1关断
  In1 : Inport
  In2 : Inport  Port=2
  Abs1 : Abs  SaturateOnIntegerOverflow=off
  Add : Sum
  Constant1 : Constant  Value=0
  Constant2 : Constant  Value=0
  Gain1 : Gain  Gain=Udc/DIODE_D1031SH.Vdc
  Gain2 : Gain  Gain=DIODE_D1031SH.Err/DIODE_D1031SH.IFQ
  Gain3 : Gain  Gain=1/Ts2
  Gain4 : Gain
  Logical Operator2 : Logic  Operator=NOT  AllPortsSameDT=off  OutDataTypeStr=boolean
  Logical Operator3 : Logic  AllPortsSameDT=off  OutDataTypeStr=boolean
  Logical Operator4 : Logic  AllPortsSameDT=off  OutDataTypeStr=boolean
  Logical Operator5 : Logic  Operator=NOT  AllPortsSameDT=off  OutDataTypeStr=boolean
  Pulse Generator : DiscretePulseGenerator  PulseType=Time based  Period=Ts2  PulseWidth=5
  Saturation : Saturate  UpperLimit=5500  LowerLimit=0
  Saturation1 : Saturate  UpperLimit=100  LowerLimit=0
  Switch2 : Switch  Criteria=u2 > Threshold  SaturateOnIntegerOverflow=off  InputSameDT=off
  Switch3 : Switch  Criteria=u2 > Threshold  SaturateOnIntegerOverflow=off  InputSameDT=off
  Switch4 : Switch  Criteria=u2 > Threshold  SaturateOnIntegerOverflow=off  InputSameDT=off
  Unit Delay{,1..3} (4 alike) : UnitDelay  SampleTime=Ts1  HasFrameUpgradeWarning=on
  Out1 : Outport  VectorParamsAs1DForOutWhenUnconnected=off
  wires:
  Gain2/1 -> Saturation1/1
  Saturation/1 -> Gain2/1
  Saturation1/1 -> Switch2/1
  Gain4/1 -> Saturation/1
  Unit Delay/1 -> Logical Operator2/1
  Add/1 -> Unit Delay1/1
  In1/1 -> Gain4/1
  Gain3/1 -> Out1/1
  Unit Delay1/1 -> Switch4/1, Switch3/3
  Logical Operator4/1 -> Switch3/2, Switch4/2
  Logical Operator5/1 -> Logical Operator4/2
  Unit Delay3/1 -> Logical Operator5/1
  Unit Delay2/1 -> Switch4/3
  Switch4/1 -> Gain3/1, Unit Delay2/1
  Pulse Generator/1 -> Logical Operator4/1, Unit Delay3/1
  Constant1/1 -> Switch3/1
  Switch3/1 -> Add/2
  Constant2/1 -> Switch2/3
  Logical Operator3/1 -> Switch2/2
  Logical Operator2/1 -> Logical Operator3/2
  In2/1 -> Unit Delay/1, Logical Operator3/1
  Gain1/1 -> Abs1/1
  Switch2/1 -> Gain1/1
  Abs1/1 -> Add/1

== system power_10MW5_diode/JUNCTION LOSS and TEMP/DIODE/D1331SH/D1331SH_MAIN/Subsystem ==
  In1 : Inport
  Gain44 : Gain  Gain=DIODE_D1331SH.rF
  Gain45 : Gain  Gain=DIODE_D1331SH.VF0
  Math Function9 : Math  Operator=magnitude^2  SignedPower=on
  Mean79 : spsMeanLib/Mean  Freq=2000  Vinit=0  Ts=Ts1
  RMS9 : spsRMSLib/RMS  TrueRMS=on  Freq=2000  RMSInit=0  Ts=Ts1
  Out1 : Outport
  Out2 : Outport  Port=2
  wires:
  Gain45/1 -> Out2/1
  In1/1 -> RMS9/1, Mean79/1
  Math Function9/1 -> Gain44/1
  Mean79/1 -> Gain45/1
  Gain44/1 -> Out1/1
  RMS9/1 -> Math Function9/1

== system power_10MW5_diode/JUNCTION LOSS and TEMP/DIODE/D1331SH/D1331SH_MAIN/Subsystem1 ==
  note: 散热器热阻：水到壳
  note: 器件手册热阻：壳到结
  note: 接触热阻：散热器到壳
      | 需考虑单面散热还是双面
      | 时间常数估计的？
  In1 : Inport
  In2 : Inport  Port=2
  Add3 : Sum
  Add4 : Sum  Inputs=6
  Add5 : Sum  Inputs=+++
  Constant : Constant  Value=temp_init
  Discrete Filter1 : DiscreteFilter  Numerator=[Ts2/DIODE_D1331SH.Rth_jc1_dou_tau]  Denominator=[1 (Ts2/DIODE_D1331SH.Rth_jc1_dou_tau)-1]  SampleTime=Ts2
  Discrete Filter2 : DiscreteFilter  Numerator=[Ts2/DIODE_D1331SH.Rth_jc2_dou_tau]  Denominator=[1 (Ts2/DIODE_D1331SH.Rth_jc2_dou_tau)-1]  SampleTime=Ts2
  Discrete Filter3 : DiscreteFilter  Numerator=[Ts2/DIODE_D1331SH.Rth_jc3_dou_tau]  Denominator=[1 (Ts2/DIODE_D1331SH.Rth_jc3_dou_tau)-1]  SampleTime=Ts2
  Discrete Filter4 : DiscreteFilter  Numerator=[Ts2/DIODE_D1331SH.Rth_jc4_dou_tau]  Denominator=[1 (Ts2/DIODE_D1331SH.Rth_jc4_dou_tau)-1]  SampleTime=Ts2
  Discrete Filter5 : DiscreteFilter  Numerator=[Ts2/DIODE_D1331SH.Rth_ch_dou_tau]  Denominator=[1 (Ts2/DIODE_D1331SH.Rth_ch_dou_tau)-1]  SampleTime=Ts2
  Discrete Filter6 : DiscreteFilter  Numerator=[Ts2/DIODE_D1331SH.Rth_jc5_dou_tau]  Denominator=[1 (Ts2/DIODE_D1331SH.Rth_jc5_dou_tau)-1]  SampleTime=Ts2
  Discrete Filter9 : DiscreteFilter  Numerator=[Ts2/Rth_h_tau]  Denominator=[1 (Ts2/Rth_h_tau)-1]  SampleTime=Ts2
  Gain1 : Gain  Gain=DIODE_D1331SH.Rth_jc1_dou
  Gain2 : Gain  Gain=DIODE_D1331SH.Rth_jc2_dou
  Gain3 : Gain  Gain=DIODE_D1331SH.Rth_jc3_dou
  Gain4 : Gain  Gain=DIODE_D1331SH.Rth_jc4_dou
  Gain5 : Gain  Gain=DIODE_D1331SH.Rth_ch_dou
  Gain6 : Gain  Gain=DIODE_D1331SH.Rth_jc5_dou
  Gain9 : Gain  Gain=Rth_h
  Out1 : Outport  VectorParamsAs1DForOutWhenUnconnected=off
  wires:
  Discrete Filter4/1 -> Add4/5
  Gain4/1 -> Discrete Filter4/1
  In1/1 -> Add3/1
  Gain2/1 -> Discrete Filter2/1
  Discrete Filter2/1 -> Add4/3
  Add4/1 -> Add5/2
  In2/1 -> Add3/2
  Constant/1 -> Add5/3
  Gain1/1 -> Discrete Filter1/1
  Add5/1 -> Out1/1
  Discrete Filter1/1 -> Add4/2
  Gain5/1 -> Discrete Filter5/1
  Discrete Filter5/1 -> Add4/1
  Gain3/1 -> Discrete Filter3/1
  Discrete Filter3/1 -> Add4/4
  Add3/1 -> Gain3/1, Gain5/1, Gain6/1, Gain4/1, Gain9/1, Gain1/1, Gain2/1
  Gain9/1 -> Discrete Filter9/1
  Discrete Filter9/1 -> Add5/1
  Gain6/1 -> Discrete Filter6/1
  Discrete Filter6/1 -> Add4/6

== system power_10MW5_diode/JUNCTION LOSS and TEMP/DIODE/D1331SH/D1331SH_MAIN/Subsystem2 ==
  note: 用于判断D1关断时刻，电流为负时，T3开通就意味着D1关断
  In1 : Inport
  In2 : Inport  Port=2
  Abs1 : Abs  SaturateOnIntegerOverflow=off
  Add : Sum
  Constant1 : Constant  Value=0
  Constant2 : Constant  Value=0
  Gain1 : Gain  Gain=Udc/DIODE_D1331SH.Vdc
  Gain2 : Gain  Gain=DIODE_D1331SH.Err/DIODE_D1331SH.IFQ
  Gain3 : Gain  Gain=1/Ts2
  Gain4 : Gain
  Logical Operator2 : Logic  Operator=NOT  AllPortsSameDT=off  OutDataTypeStr=boolean
  Logical Operator3 : Logic  AllPortsSameDT=off  OutDataTypeStr=boolean
  Logical Operator4 : Logic  AllPortsSameDT=off  OutDataTypeStr=boolean
  Logical Operator5 : Logic  Operator=NOT  AllPortsSameDT=off  OutDataTypeStr=boolean
  Pulse Generator : DiscretePulseGenerator  PulseType=Time based  Period=Ts2  PulseWidth=5
  Saturation : Saturate  UpperLimit=5500  LowerLimit=0
  Saturation1 : Saturate  UpperLimit=100  LowerLimit=0
  Switch2 : Switch  Criteria=u2 > Threshold  SaturateOnIntegerOverflow=off  InputSameDT=off
  Switch3 : Switch  Criteria=u2 > Threshold  SaturateOnIntegerOverflow=off  InputSameDT=off
  Switch4 : Switch  Criteria=u2 > Threshold  SaturateOnIntegerOverflow=off  InputSameDT=off
  Unit Delay{,1..3} (4 alike) : UnitDelay  SampleTime=Ts1  HasFrameUpgradeWarning=on
  Out1 : Outport  VectorParamsAs1DForOutWhenUnconnected=off
  wires:
  Abs1/1 -> Add/1
  Switch2/1 -> Gain1/1
  Gain1/1 -> Abs1/1
  In2/1 -> Logical Operator3/1, Unit Delay/1
  Logical Operator2/1 -> Logical Operator3/2
  Logical Operator3/1 -> Switch2/2
  Constant2/1 -> Switch2/3
  Switch3/1 -> Add/2
  Constant1/1 -> Switch3/1
  Pulse Generator/1 -> Unit Delay3/1, Logical Operator4/1
  Switch4/1 -> Unit Delay2/1, Gain3/1
  Unit Delay2/1 -> Switch4/3
  Unit Delay3/1 -> Logical Operator5/1
  Logical Operator5/1 -> Logical Operator4/2
  Logical Operator4/1 -> Switch4/2, Switch3/2
  Unit Delay1/1 -> Switch3/3, Switch4/1
  Gain3/1 -> Out1/1
  In1/1 -> Gain4/1
  Add/1 -> Unit Delay1/1
  Unit Delay/1 -> Logical Operator2/1
  Gain4/1 -> Saturation/1
  Saturation1/1 -> Switch2/1
  Saturation/1 -> Gain2/1
  Gain2/1 -> Saturation1/1

== system power_10MW5_diode/JUNCTION LOSS and TEMP/DIODE/D1331SH/D1331SH_MAIN/Subsystem29 ==
  note: 用于判断D1关断时刻，电流为负时，T3开通就意味着D1关断
  In1 : Inport
  In2 : Inport  Port=2
  Abs1 : Abs  SaturateOnIntegerOverflow=off
  Add : Sum
  Constant1 : Constant  Value=0
  Constant2 : Constant  Value=0
  Gain1 : Gain  Gain=Udc/DIODE_D1331SH.Vdc
  Gain2 : Gain  Gain=DIODE_D1331SH.Err/DIODE_D1331SH.IFQ
  Gain3 : Gain  Gain=1/Ts2
  Gain4 : Gain
  Logical Operator2 : Logic  Operator=NOT  AllPortsSameDT=off  OutDataTypeStr=boolean
  Logical Operator3 : Logic  AllPortsSameDT=off  OutDataTypeStr=boolean
  Logical Operator4 : Logic  AllPortsSameDT=off  OutDataTypeStr=boolean
  Logical Operator5 : Logic  Operator=NOT  AllPortsSameDT=off  OutDataTypeStr=boolean
  Pulse Generator : DiscretePulseGenerator  PulseType=Time based  Period=Ts2  PulseWidth=5
  Saturation : Saturate  UpperLimit=5500  LowerLimit=0
  Saturation1 : Saturate  UpperLimit=100  LowerLimit=0
  Switch2 : Switch  Criteria=u2 > Threshold  SaturateOnIntegerOverflow=off  InputSameDT=off
  Switch3 : Switch  Criteria=u2 > Threshold  SaturateOnIntegerOverflow=off  InputSameDT=off
  Switch4 : Switch  Criteria=u2 > Threshold  SaturateOnIntegerOverflow=off  InputSameDT=off
  Unit Delay{,1..3} (4 alike) : UnitDelay  SampleTime=Ts1  HasFrameUpgradeWarning=on
  Out1 : Outport  VectorParamsAs1DForOutWhenUnconnected=off
  wires:
  Gain2/1 -> Saturation1/1
  Saturation/1 -> Gain2/1
  Saturation1/1 -> Switch2/1
  Gain4/1 -> Saturation/1
  Unit Delay/1 -> Logical Operator2/1
  Add/1 -> Unit Delay1/1
  In1/1 -> Gain4/1
  Gain3/1 -> Out1/1
  Unit Delay1/1 -> Switch4/1, Switch3/3
  Logical Operator4/1 -> Switch3/2, Switch4/2
  Logical Operator5/1 -> Logical Operator4/2
  Unit Delay3/1 -> Logical Operator5/1
  Unit Delay2/1 -> Switch4/3
  Switch4/1 -> Gain3/1, Unit Delay2/1
  Pulse Generator/1 -> Logical Operator4/1, Unit Delay3/1
  Constant1/1 -> Switch3/1
  Switch3/1 -> Add/2
  Constant2/1 -> Switch2/3
  Logical Operator3/1 -> Switch2/2
  Logical Operator2/1 -> Logical Operator3/2
  In2/1 -> Unit Delay/1, Logical Operator3/1
  Gain1/1 -> Abs1/1
  Switch2/1 -> Gain1/1
  Abs1/1 -> Add/1

== system power_10MW5_diode/JUNCTION LOSS and TEMP/DIODE/D1331SH/D1331SH_MAIN/Subsystem3 ==
  In1 : Inport
  Abs1 : Abs  SaturateOnIntegerOverflow=off
  Add : Sum
  Add1 : Sum
  Constant : Constant
  Constant1 : Constant  Value=0
  Constant2 : Constant  Value=0
  Data Type Conversion : DataTypeConversion  OutDataTypeStr=boolean  SaturateOnIntegerOverflow=off  RndMeth=Floor
  Data Type Conversion1 : DataTypeConversion  SaturateOnIntegerOverflow=off  RndMeth=Floor
  Gain : Gain  Gain=-1
  Gain2 : Gain  Gain=Udc/DIODE_D1331SH.Vdc
  Gain3 : Gain  Gain=1/Ts2
  Gain6 : Gain
  Gain8 : Gain  Gain=DIODE_D1331SH.Err/DIODE_D1331SH.IFQ
  Logical Operator2 : Logic  Operator=NOT  AllPortsSameDT=off  OutDataTypeStr=boolean
  Logical Operator4 : Logic  AllPortsSameDT=off  OutDataTypeStr=boolean
  Logical Operator5 : Logic  Operator=NOT  AllPortsSameDT=off  OutDataTypeStr=boolean
  Pulse Generator : DiscretePulseGenerator  PulseType=Time based  Period=Ts2  PulseWidth=5
  Saturation2 : Saturate  UpperLimit=5500  LowerLimit=0
  Saturation3 : Saturate  UpperLimit=100  LowerLimit=0
  Scope1 : Scope  NumInputPorts=3
  Scope7 : Scope  NumInputPorts=2
  Switch2 : Switch  Criteria=u2 > Threshold  Threshold=-1  SaturateOnIntegerOverflow=off  InputSameDT=off
  Switch3 : Switch  Criteria=u2 > Threshold  SaturateOnIntegerOverflow=off  InputSameDT=off
  Switch4 : Switch  Criteria=u2 > Threshold  SaturateOnIntegerOverflow=off  InputSameDT=off
  Terminator : Terminator
  Unit Delay{,1..3} (4 alike) : UnitDelay  SampleTime=1e-6  HasFrameUpgradeWarning=on
  Out1 : Outport  VectorParamsAs1DForOutWhenUnconnected=off
  wires:
  Saturation3/1 -> Terminator/1
  Gain8/1 -> Saturation3/1
  Saturation2/1 -> Gain8/1
  Gain6/1 -> Saturation2/1
  Constant/1 -> Switch2/1
  Data Type Conversion1/1 -> Gain/1
  Gain/1 -> Switch2/2
  Add1/1 -> Data Type Conversion1/1
  Data Type Conversion/1 -> Unit Delay/1, Add1/1
  Logical Operator2/1 -> Add1/2
  Unit Delay/1 -> Logical Operator2/1
  Abs1/1 -> Add/1
  Switch2/1 -> Gain2/1
  Gain2/1 -> Abs1/1, Scope1/1
  In1/1 -> Gain6/1, Data Type Conversion/1
  Constant2/1 -> Switch2/3
  Switch3/1 -> Add/2
  Constant1/1 -> Switch3/1
  Pulse Generator/1 -> Unit Delay3/1, Logical Operator4/1
  Switch4/1 -> Scope7/2, Unit Delay2/1, Gain3/1
  Unit Delay2/1 -> Switch4/3
  Unit Delay3/1 -> Logical Operator5/1
  Logical Operator5/1 -> Logical Operator4/2
  Logical Operator4/1 -> Scope1/3, Switch4/2, Switch3/2
  Unit Delay1/1 -> Scope7/1, Switch3/3, Switch4/1
  Gain3/1 -> Out1/1
  Add/1 -> Scope1/2, Unit Delay1/1

== system power_10MW5_diode/JUNCTION LOSS and TEMP/DIODE/D1331SH/D1331SH_MAIN/Subsystem34 ==
  In1 : Inport
  In2 : Inport  Port=2
  In3 : Inport  Port=3
  Abs1 : Abs  SaturateOnIntegerOverflow=off
  Add : Sum
  Constant1 : Constant  Value=0
  Constant2 : Constant  Value=0
  Gain2 : Gain  Gain=Udc/DIODE_204520.Vdc
  Gain3 : Gain  Gain=1/Ts2
  Gain4 : Gain
  Gain8 : Gain  Gain=DIODE_D1331SH.Err/DIODE_D1331SH.IFQ
  Logical Operator1 : Logic  Operator=NOT  AllPortsSameDT=off  OutDataTypeStr=boolean
  Logical Operator11 : Logic  Operator=OR  AllPortsSameDT=off  OutDataTypeStr=boolean
  Logical Operator2 : Logic  Operator=NOT  AllPortsSameDT=off  OutDataTypeStr=boolean
  Logical Operator3 : Logic  AllPortsSameDT=off  OutDataTypeStr=boolean
  Logical Operator4 : Logic  AllPortsSameDT=off  OutDataTypeStr=boolean
  Logical Operator5 : Logic  Operator=NOT  AllPortsSameDT=off  OutDataTypeStr=boolean
  Logical Operator6 : Logic  AllPortsSameDT=off  OutDataTypeStr=boolean
  Pulse Generator : DiscretePulseGenerator  PulseType=Time based  Period=Ts2  PulseWidth=5
  Saturation : Saturate  UpperLimit=5500  LowerLimit=0
  Saturation1 : Saturate  UpperLimit=100  LowerLimit=0
  Scope1 : Scope  NumInputPorts=3
  Scope7 : Scope  NumInputPorts=2
  Switch2 : Switch  Criteria=u2 > Threshold  SaturateOnIntegerOverflow=off  InputSameDT=off
  Switch3 : Switch  Criteria=u2 > Threshold  SaturateOnIntegerOverflow=off  InputSameDT=off
  Switch4 : Switch  Criteria=u2 > Threshold  SaturateOnIntegerOverflow=off  InputSameDT=off
  Unit Delay{,1..4} (5 alike) : UnitDelay  SampleTime=1e-6  HasFrameUpgradeWarning=on
  Out1 : Outport  VectorParamsAs1DForOutWhenUnconnected=off
  wires:
  Gain8/1 -> Saturation1/1
  Saturation/1 -> Gain8/1
  Logical Operator3/1 -> Logical Operator11/1
  Logical Operator11/1 -> Switch2/2
  Logical Operator1/1 -> Logical Operator6/2
  Logical Operator6/1 -> Logical Operator11/2
  Unit Delay4/1 -> Logical Operator1/1
  In3/1 -> Logical Operator6/1, Unit Delay4/1
  Saturation1/1 -> Switch2/1
  Gain4/1 -> Saturation/1
  Unit Delay/1 -> Logical Operator2/1
  Add/1 -> Unit Delay1/1, Scope1/2
  In1/1 -> Gain4/1
  Gain3/1 -> Out1/1
  Unit Delay1/1 -> Switch3/3, Switch4/1, Scope7/1
  Logical Operator4/1 -> Scope1/3, Switch3/2, Switch4/2
  Logical Operator5/1 -> Logical Operator4/2
  Unit Delay3/1 -> Logical Operator5/1
  Unit Delay2/1 -> Switch4/3
  Switch4/1 -> Unit Delay2/1, Gain3/1, Scope7/2
  Pulse Generator/1 -> Logical Operator4/1, Unit Delay3/1
  Constant1/1 -> Switch3/1
  Switch3/1 -> Add/2
  Constant2/1 -> Switch2/3
  Logical Operator2/1 -> Logical Operator3/2
  In2/1 -> Unit Delay/1, Logical Operator3/1
  Gain2/1 -> Scope1/1, Abs1/1
  Switch2/1 -> Gain2/1
  Abs1/1 -> Add/1

== system power_10MW5_diode/JUNCTION LOSS and TEMP/DIODE/D1331SH/D1331SH_MAIN/Subsystem4 ==
  In1 : Inport
  Gain44 : Gain  Gain=DIODE_D1331SH.rF
  Gain45 : Gain  Gain=DIODE_D1331SH.VF0
  Math Function9 : Math  Operator=magnitude^2  SignedPower=on
  Mean79 : spsMeanLib/Mean  Freq=2000  Vinit=0  Ts=Ts1
  RMS9 : spsRMSLib/RMS  TrueRMS=on  Freq=2000  RMSInit=0  Ts=Ts1
  Out1 : Outport
  Out2 : Outport  Port=2
  wires:
  Gain45/1 -> Out2/1
  In1/1 -> RMS9/1, Mean79/1
  Math Function9/1 -> Gain44/1
  Mean79/1 -> Gain45/1
  Gain44/1 -> Out1/1
  RMS9/1 -> Math Function9/1

== system power_10MW5_diode/JUNCTION LOSS and TEMP/DIODE/D1331SH/D1331SH_MAIN/Subsystem5 ==
  note: 接触热阻：散热器到壳
      | 需考虑单面散热还是双面
      | 时间常数估计的？
  note: 器件手册热阻：壳到结
  note: 散热器热阻：水到壳
  In1 : Inport
  In2 : Inport  Port=2
  Add3 : Sum
  Add4 : Sum  Inputs=6
  Add5 : Sum  Inputs=+++
  Constant : Constant  Value=temp_init
  Discrete Filter1 : DiscreteFilter  Numerator=[Ts2/DIODE_D1331SH.Rth_jc1_dou_tau]  Denominator=[1 (Ts2/DIODE_D1331SH.Rth_jc1_dou_tau)-1]  SampleTime=Ts2
  Discrete Filter2 : DiscreteFilter  Numerator=[Ts2/DIODE_D1331SH.Rth_jc2_dou_tau]  Denominator=[1 (Ts2/DIODE_D1331SH.Rth_jc2_dou_tau)-1]  SampleTime=Ts2
  Discrete Filter3 : DiscreteFilter  Numerator=[Ts2/DIODE_D1331SH.Rth_jc3_dou_tau]  Denominator=[1 (Ts2/DIODE_D1331SH.Rth_jc3_dou_tau)-1]  SampleTime=Ts2
  Discrete Filter4 : DiscreteFilter  Numerator=[Ts2/DIODE_D1331SH.Rth_jc4_dou_tau]  Denominator=[1 (Ts2/DIODE_D1331SH.Rth_jc4_dou_tau)-1]  SampleTime=Ts2
  Discrete Filter5 : DiscreteFilter  Numerator=[Ts2/DIODE_D1331SH.Rth_ch_dou_tau]  Denominator=[1 (Ts2/DIODE_D1331SH.Rth_ch_dou_tau)-1]  SampleTime=Ts2
  Discrete Filter6 : DiscreteFilter  Numerator=[Ts2/DIODE_D1331SH.Rth_jc5_dou_tau]  Denominator=[1 (Ts2/DIODE_D1331SH.Rth_jc5_dou_tau)-1]  SampleTime=Ts2
  Discrete Filter9 : DiscreteFilter  Numerator=[Ts2/Rth_h_tau]  Denominator=[1 (Ts2/Rth_h_tau)-1]  SampleTime=Ts2
  Gain1 : Gain  Gain=DIODE_D1331SH.Rth_jc1_dou
  Gain2 : Gain  Gain=DIODE_D1331SH.Rth_jc2_dou
  Gain3 : Gain  Gain=DIODE_D1331SH.Rth_jc3_dou
  Gain4 : Gain  Gain=DIODE_D1331SH.Rth_jc4_dou
  Gain5 : Gain  Gain=DIODE_D1331SH.Rth_ch_dou
  Gain6 : Gain  Gain=DIODE_D1331SH.Rth_jc5_dou
  Gain9 : Gain  Gain=Rth_h
  Out1 : Outport  VectorParamsAs1DForOutWhenUnconnected=off
  wires:
  Discrete Filter6/1 -> Add4/6
  Gain6/1 -> Discrete Filter6/1
  Discrete Filter9/1 -> Add5/1
  Gain9/1 -> Discrete Filter9/1
  Add3/1 -> Gain2/1, Gain1/1, Gain9/1, Gain4/1, Gain6/1, Gain5/1, Gain3/1
  Discrete Filter3/1 -> Add4/4
  Gain3/1 -> Discrete Filter3/1
  Discrete Filter5/1 -> Add4/1
  Gain5/1 -> Discrete Filter5/1
  Discrete Filter1/1 -> Add4/2
  Add5/1 -> Out1/1
  Gain1/1 -> Discrete Filter1/1
  Constant/1 -> Add5/3
  In2/1 -> Add3/2
  Add4/1 -> Add5/2
  Discrete Filter2/1 -> Add4/3
  Gain2/1 -> Discrete Filter2/1
  In1/1 -> Add3/1
  Gain4/1 -> Discrete Filter4/1
  Discrete Filter4/1 -> Add4/5
